simulink model "stage10"  (Simulink 7.7)
settings: Solver=ode45  StartTime=0.0  StopTime=0.1  RelTol=1e-3
undefined symbols (not defined in the file): Acid, idx_data, iv_data, Lead
libraries: powerlib x16, simulink x4, fl_lib x4, nesl_utility x3, electricdrivelib x2, elec_lib x2, powerlib_extras x1
settings Model: Creator=Vikas  LastModifiedBy=HASANTH

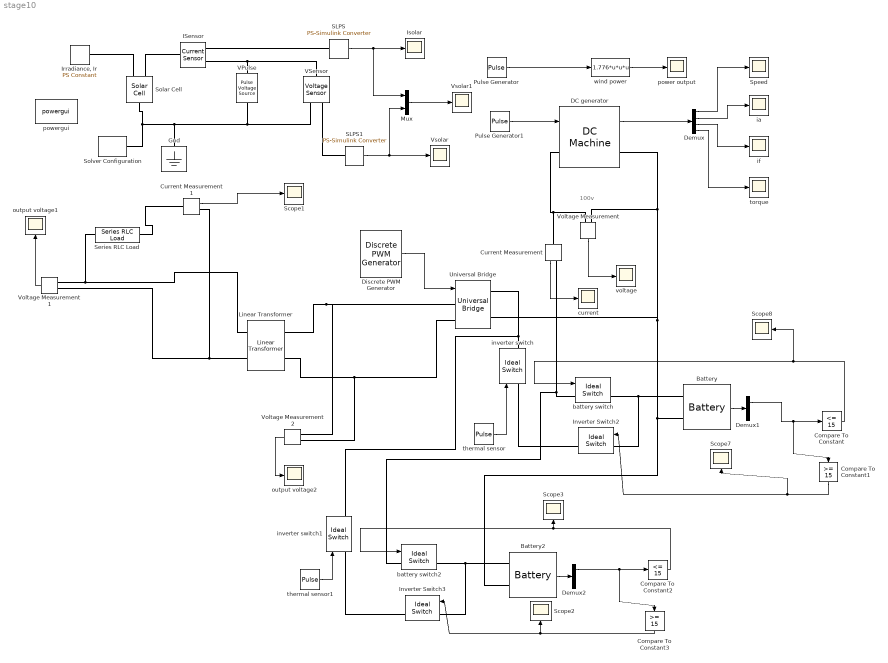
== system stage10 ==
  note: 100v
  Battery : electricdrivelib/Extra Sources/Battery  SystemSampleTime=-1  BatType=Lead-Acid  ShowDetailedParameters=off  NomV=15  NomQ=60  SOC=100  PresetModel=on  MaxQ=62.5  FullV=16.3322  Dis_rate=12  R=0.0025  Normal_OP=18.6167  expZone="[15.2714          0.2]"  Dis_Char=off  current=[6.5 13 32.5]  Units=Time  Batt_Tr=5
  Battery2 : electricdrivelib/Extra Sources/Battery  SystemSampleTime=-1  BatType=Lead-Acid  ShowDetailedParameters=off  NomV=15  NomQ=60  SOC=100  PresetModel=on  MaxQ=62.5  FullV=16.3322  Dis_rate=12  R=0.0025  Normal_OP=18.6167  expZone="[15.2714          0.2]"  Dis_Char=off  current=[6.5 13 32.5]  Units=Time  Batt_Tr=5
  Compare To Constant : simulink/Logic and Bit Operations/Compare To Constant  SystemSampleTime=-1  relop=<=  const=15  LogicOutDataTypeMode=uint8
  Compare To Constant1 : simulink/Logic and Bit Operations/Compare To Constant  SystemSampleTime=-1  relop=>=  const=15  LogicOutDataTypeMode=uint8
  Compare To Constant2 : simulink/Logic and Bit Operations/Compare To Constant  SystemSampleTime=-1  relop=<=  const=15  LogicOutDataTypeMode=uint8
  Compare To Constant3 : simulink/Logic and Bit Operations/Compare To Constant  SystemSampleTime=-1  relop=>=  const=15  LogicOutDataTypeMode=uint8
  Current Measurement : powerlib/Measurements/Current Measurement  SystemSampleTime=-1  PhasorSimulation=off  OutputType=Complex  PSBequivalent=0
  Current Measurement1 : powerlib/Measurements/Current Measurement  SystemSampleTime=-1  PhasorSimulation=off  OutputType=Complex  PSBequivalent=0
  DC generator : powerlib/Machines/DC Machine  SystemSampleTime=-1  PresetModel=No  MechanicalLoad=Speed w  FieldType=Permanent magnet  ShowDetailedParameters=on  RLa="[ 2  0.012]"  RLf="[ 240  120]"  Laf=1.8  MachineConstant=Back-emf constant (V/rpm)  Ke=3  Kt=3.18  J=1  Bm=0  Tf=0  w0=1  Ifinit=1  TsPowergui=0  TsBlock=-1
      settings: AttributesFormatString=\n
  Demux : Demux
  Demux1 : Demux  Outputs=3
  Demux2 : Demux  Outputs=3
  Discrete PWM Generator : powerlib_extras/Discrete  Control Blocks/Discrete PWM Generator  SystemSampleTime=-1  GeneratorMode="2-arm  bridge (4 pulses)"  Fc=1080  Ts=5e-6  Internal=on  mIndex=0.4  Freq=50  Phase=0
  Gnd : fl_lib/Electrical/Electrical Elements/Electrical Reference  SystemSampleTime=-1  i_Log=off  LocalVarNames=|i  LocalVarDescs=|i  LocalVarLogging=[]
  ISensor : fl_lib/Electrical/Electrical Sensors/Current Sensor  SystemSampleTime=-1  i1_Log=off  v1_Log=off  LocalVarNames=|i1|v1  LocalVarDescs=|i1|v1  LocalVarLogging=[0 0]
  Inverter Switch2 : powerlib/Power Electronics/Ideal Switch  SystemSampleTime=-1  Ron=0.001  Lon=0  IC=0  Rs=1e5  Cs=inf  Measurements=on
  Inverter Switch3 : powerlib/Power Electronics/Ideal Switch  SystemSampleTime=-1  Ron=0.001  Lon=0  IC=0  Rs=1e5  Cs=inf  Measurements=on
  "Irradiance, Ir" : fl_lib/Physical Signals/Sources/PS Constant  SystemSampleTime=-1  constant=1000  LocalVarLogging=[]
  Isolar : Scope
      settings: TimeRange=1  YMin=2  YMax=8  SaveName=Io
  Linear Transformer : powerlib/Elements/Linear Transformer  PhysicalDomain=powersysdomain  SubClassName=unknown  LeftPortType=p1  RightPortType=p1  LConnTagsString=a|b  RConnTagsString=A|B  UNITS=pu  NominalPower=[ 875 50 ]  winding1=[15 0.002 0]  winding2=[240 0.002 0.0]  ThreeWindings=off  winding3=[3.15e+005 0.002 0.08]  RmLm=[500 500]  Measurements=None  DataType=off
  Mux : Mux  Inputs=2
  Pulse Generator : DiscretePulseGenerator  PulseType=Time based  Amplitude=3.84  Period=10  PulseWidth=50
  Pulse Generator1 : DiscretePulseGenerator  PulseType=Time based  Amplitude=5.3  Period=10  PulseWidth=50
  SLPS : nesl_utility/PS-Simulink Converter  SystemSampleTime=-1  PhysicalDomain=network_engine_domain  LeftPortType=input  RightPortType=output  SubClassName=ps_output  Unit=1  AffineConversion=off
  SLPS1 : nesl_utility/PS-Simulink Converter  SystemSampleTime=-1  PhysicalDomain=network_engine_domain  LeftPortType=input  RightPortType=output  SubClassName=ps_output  Unit=1  AffineConversion=off
  Scope{1..3,7..8} (5 alike) : Scope
      Scope1 settings: TimeRange=0.1  YMin=-1.1  YMax=1.2  SaveName=ScopeData11
      Scope2 settings: TimeRange=0.1  YMin=0.95  YMax=1.05  SaveName=ScopeData5
      Scope3 settings: TimeRange=0.02  YMin=0.95  YMax=1.05  SaveName=ScopeData10
      Scope7 settings: TimeRange=0.1  YMin=0.95  YMax=1.05  SaveName=ScopeData7
      Scope8 settings: TimeRange=0.02  YMin=0.95  YMax=1.05  SaveName=ScopeData9
  Series RLC Load : powerlib/Elements/Series RLC Load  PhysicalDomain=powersysdomain  SubClassName=unknown  LeftPortType=p1  RightPortType=p1  LConnTagsString=a  RConnTagsString=__new0  NominalVoltage=230  NominalFrequency=50  ActivePower=500  InductivePower=200  CapacitivePower=300  Setx0=off  InitialVoltage=0  SetiL0=off  InitialCurrent=0  Measurements=None
  Solar Cell : elec_lib/Sources/Solar Cell  SystemSampleTime=-1  prm=1  Isc=0.93 A  Voc=40 V  Is=1e-06 A  Is2=0 A  Iph=7.34 A  Ir0=1000 W/m^2  ec=1.5  N2=2  Rs=0 Ohm  Rp=Inf Ohm  TIPH1=0 1/K  EG=1.11 eV  TXIS1=3  TXIS2=3  TRS1=0  TRP1=0  TFIXED=iv_data(idx_data).temperature C  Tmeas=25 C  LocalVarLogging=[]
  Solver Configuration : nesl_utility/Solver Configuration  SystemSampleTime=-1  PhysicalDomain=network_engine_domain  LeftPortType=input  RightPortType=generic  SubClassName=solver  Accelerate=off  Profile=off  ResidualTolerance=1e-9  MaxNonlinIter=3  MaxModeIter=2  DoFixedCost=off  UseLocalSampling=off  DoDC=off  LinearAlgebra=Sparse  LocalSolverSampleTime=.001  LocalSolverChoice=NE_BACKWARD_EULER_ADVANCER  UseLocalSolver=off
  Speed : Scope
  Universal Bridge : powerlib/Power Electronics/Universal Bridge  SystemSampleTime=-1  Arms=2  SnubberResistance=1e5  SnubberCapacitance=inf  Device=MOSFET / Diodes  Ron=1e-3  Lon=0  ForwardVoltages="[  0  0  ]"  ForwardVoltage=0  GTOparameters=[ 10e-6 , 20e-6 ]  IGBTparameters=[ 1e-6 , 2e-6 ]  Measurements=None  Measurements_2=None  converterType=Rectifier
  VPulse : elec_lib/Additional Components/SPICE-Compatible Components/Sources/Pulse Voltage Source  SystemSampleTime=-1  V1=0 V  V2=iv_data(idx_data).v(end) V  TD=0 s  TR=1 s  TF=0 s  PW=Inf s  PER=Inf s  voltage_Log=off  LocalVarNames=|voltage  LocalVarDescs=|Voltage (V)  LocalVarLogging=0
  VSensor : fl_lib/Electrical/Electrical Sensors/Voltage Sensor  SystemSampleTime=-1  i1_Log=off  v1_Log=off  LocalVarNames=|i1|v1  LocalVarDescs=|i1|v1  LocalVarLogging=[0 0]
  Voltage Measurement : powerlib/Measurements/Voltage Measurement  SystemSampleTime=-1  PhasorSimulation=off  OutputType=Complex  PSBequivalent=0
  Voltage Measurement1 : powerlib/Measurements/Voltage Measurement  SystemSampleTime=-1  PhasorSimulation=off  OutputType=Complex  PSBequivalent=0
  Voltage Measurement2 : powerlib/Measurements/Voltage Measurement  SystemSampleTime=-1  PhasorSimulation=off  OutputType=Complex  PSBequivalent=0
  Vsolar : Scope
      settings: TimeRange=1  YMin=0  YMax=0.8  SaveName=Vo
  Vsolar1 : Scope
      settings: TimeRange=1  YMin=0  YMax=0.8  SaveName=Vo1
  battery switch : powerlib/Power Electronics/Ideal Switch  SystemSampleTime=-1  Ron=0.001  Lon=0  IC=0  Rs=1e5  Cs=inf  Measurements=on
  battery switch2 : powerlib/Power Electronics/Ideal Switch  SystemSampleTime=-1  Ron=0.001  Lon=0  IC=0  Rs=1e5  Cs=inf  Measurements=on
  current : Scope
      settings: TimeRange=0.04  YMin=16.1786  YMax=16.1788  SaveName=ScopeData6
  ia : Scope
      settings: YMin=-0.023  YMax=0
  if : Scope
      settings: SaveName=ScopeData2
  inverter switch : powerlib/Power Electronics/Ideal Switch  SystemSampleTime=-1  Ron=0.001  Lon=0  IC=0  Rs=1e5  Cs=inf  Measurements=on
  inverter switch1 : powerlib/Power Electronics/Ideal Switch  SystemSampleTime=-1  Ron=0.001  Lon=0  IC=0  Rs=1e5  Cs=inf  Measurements=on
  output voltage1 : Scope
      settings: YMin=-275  YMax=275  SaveName=ScopeData12
  output voltage2 : Scope
      settings: YMin=-17.5  YMax=17.5  SaveName=ScopeData8
  power output : Scope
      settings: TimeRange=0.1  YMin=265.673  YMax=293.639  SaveName=ScopeData13
  powergui : powerlib/powergui  Priority=1  SystemSampleTime=-1  SimulationMode=Continuous  SampleTime=50e-6  frequency=60  SPID=off  DisableSnubberDevices=off  DisableRonSwitches=off  DisableVfSwitches=off  SwTol=0  Interpol=off  DisplayEquations=off  FunctionMessages=off  frequencyindice=0  Pbase=100e6  ErrMax=1e-4  Iterations=50  UnitsV=kV  UnitsW=MW  echomessages=off  HookPort=off  EnableUseOfTLC=off  x0status=steady  RestoreLinks=no  ResistiveCurrentMeasurement=off  Frange=[0:2:500]  Ylog=off  Xlog=on  ShowGrid=off  save=off  variable=ZData  structure=ScopeData8  ZoomFFT=off  StartTime=0.0  cycles=1  DisplayStyle=1  fundamental=60  FreqAxis=off  MaxFrequency=1000  frequencyindicesteady=1  RmsSteady=1  display=off  Ts=0  methode=off
  thermal sensor : DiscretePulseGenerator  PulseType=Time based  Period=14400  PulseWidth=50
  thermal sensor1 : DiscretePulseGenerator  PulseType=Time based  Period=14400  PulseWidth=50
  torque : Scope
      settings: SaveName=ScopeData3
  voltage : Scope
      settings: TimeRange=0.04  YMin=0.0164395  YMax=0.0164505  SaveName=ScopeData4
  "wind power " : Fcn  Expr=1.776*u*u*u
  wires:
  DC generator/1 -> Demux/1
  Demux/1 -> Speed/1
  Demux/2 -> ia/1
  Demux/3 -> if/1
  Demux/4 -> torque/1
  Voltage Measurement/1 -> voltage/1
  Battery/1 -> Demux1/1
  Demux1/1 -> Compare To Constant/1, Compare To Constant1/1
  Compare To Constant/1 -> battery switch/1, Scope8/1
  Compare To Constant1/1 -> Inverter Switch2/1, Scope7/1
  Current Measurement/1 -> current/1
  Pulse Generator1/1 -> DC generator/1
  thermal sensor/1 -> inverter switch/1
  Pulse Generator/1 -> "wind power "/1
  "wind power "/1 -> power output/1
  Voltage Measurement1/1 -> output voltage1/1
  Voltage Measurement2/1 -> output voltage2/1
  Discrete PWM Generator/1 -> Universal Bridge/1
  Current Measurement1/1 -> Scope1/1
  Battery2/1 -> Demux2/1
  Demux2/1 -> Compare To Constant2/1, Compare To Constant3/1
  Compare To Constant2/1 -> battery switch2/1, Scope3/1
  Compare To Constant3/1 -> Inverter Switch3/1, Scope2/1
  thermal sensor1/1 -> inverter switch1/1
  SLPS1/1 -> Vsolar/1, Mux/2
  Mux/1 -> Vsolar1/1
  SLPS/1 -> Isolar/1, Mux/1
  connections:
  Battery/LConn1 -- battery switch/RConn1 -- Inverter Switch2/LConn1
  Current Measurement/LConn1 -- Voltage Measurement/LConn1 -- DC generator/LConn1
  Battery/LConn2 -- Voltage Measurement/LConn2 -- DC generator/RConn1 -- Universal Bridge/RConn2 -- Battery2/LConn2
  battery switch/LConn1 -- Current Measurement/RConn1 -- battery switch2/LConn1
  inverter switch/LConn1 -- Inverter Switch2/RConn1
  inverter switch/RConn1 -- Universal Bridge/RConn1 -- inverter switch1/RConn1
  Voltage Measurement1/LConn1 -- Linear Transformer/RConn1 -- Series RLC Load/LConn1
  Universal Bridge/LConn2 -- Linear Transformer/LConn2 -- Voltage Measurement2/LConn2
  Voltage Measurement2/LConn1 -- Linear Transformer/LConn1 -- Universal Bridge/LConn1
  Voltage Measurement1/LConn2 -- Linear Transformer/RConn2 -- Current Measurement1/RConn1
  Series RLC Load/RConn1 -- Current Measurement1/LConn1
  Inverter Switch3/LConn1 -- Battery2/LConn1 -- battery switch2/RConn1
  inverter switch1/LConn1 -- Inverter Switch3/RConn1
  Solver Configuration/RConn1 -- Solar Cell/RConn1 -- Gnd/LConn1 -- VPulse/RConn1 -- VSensor/RConn2
  VSensor/LConn1 -- ISensor/RConn2 -- VPulse/LConn1
  ISensor/RConn1 -- SLPS/LConn1
  VSensor/RConn1 -- SLPS1/LConn1
  ISensor/LConn1 -- Solar Cell/LConn2
  "Irradiance, Ir"/RConn1 -- Solar Cell/LConn1
